simulink model "Task_1_DSB"  (R2016a)
settings: Solver=VariableStepAuto  StartTime=0.0  StopTime=3  RelTol=1e-3
libraries: commanapbnd3 x2, dspsrcs4 x1
settings Model: Creator=92301  LastModifiedBy=92301

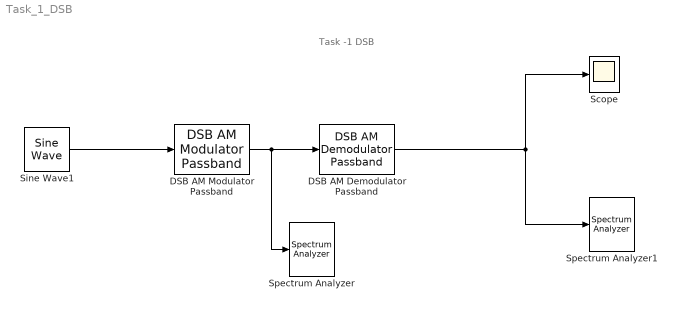
== system Task_1_DSB ==
  note: Task -1 DSB
  DSB AM Demodulator Passband : commanapbnd3/DSB AM Demodulator Passband  Fc=400  Ph=0  method=Butterworth  n=4  cf=300  Rp=0.1  Rs=50  Offset=5
  DSB AM Modulator Passband : commanapbnd3/DSB AM Modulator Passband  Fc=400  Ph=0  Offset=5
  Scope : Scope
  "Sine Wave1 " : dspsrcs4/Sine Wave  Amplitude=5  Frequency=10  Phase=0  SampleMode=Discrete  OutComplex=Real  CompMethod=Trigonometric fcn  TableSize=Speed  SampleTime=1/1000  SamplesPerFrame=1  ResetState=Restart at time zero  OutputFrames=off  dataType=double  wordLen=16  udDataType=sfix(16)  fracBitsMode=Best precision  numFracBits=15  OutDataTypeStr=double  LastOutDataTypeStr=double
  Spectrum Analyzer : SpectrumAnalyzer
  "Spectrum Analyzer1 " : SpectrumAnalyzer
  wires:
  "Sine Wave1 "/1 -> DSB AM Modulator Passband/1
  DSB AM Modulator Passband/1 -> Spectrum Analyzer/1, DSB AM Demodulator Passband/1
  DSB AM Demodulator Passband/1 -> Scope/1, "Spectrum Analyzer1 "/1
